simulink model "MHH_BUOI2_bai3"  (R2020b)
settings: Solver=VariableStepAuto  StartTime=0.0  StopTime=Sim_Time  RelTol=1e-3
values from neighbouring files (symbols this model uses):
  Cn = 8280    [Bai3_4.mat]
  I = 2.3    [Bai3_4.mat]
  OCV = [2.4 2.86404 3.33456 3.47124 3.5586 3.62364 3.6762 3.72036 3.7584 3.7902 3.81708 3.83568 ... (101 elements, 101x1)]    [Bai3_4.mat]    (also in bai4.mat)
  R_Discharge = [0.14 0.129 0.12383 0.09468 0.08038 0.07532 0.07257 0.07059 0.06894 0.06707 0.06498 0.06256 ... (101 elements, 101x1)]    [Bai3_4.mat]
  SOC = [0 0.01 0.02 0.03 0.04 0.05 0.06 0.07 0.08 0.09 0.1 0.11 ... (101 elements, 101x1)]    [Bai3_4.mat]    (also in bai4.mat)
settings Model: Creator=John Andrew  LastModifiedBy=John Andrew

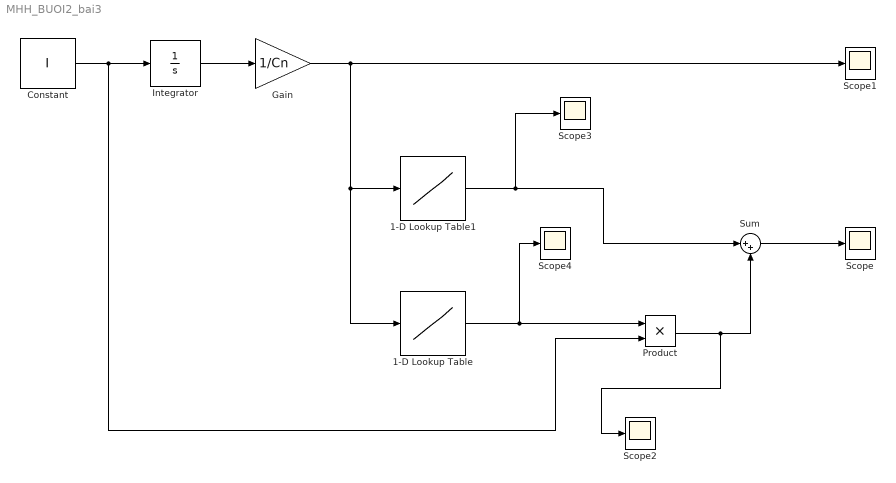
== system MHH_BUOI2_bai3 ==
  1-D Lookup Table : Lookup_n-D  NumberOfTableDimensions=1  BreakpointsForDimension1=SOC  Table=R_Discharge  InternalRulePriority=Speed  RndMeth=Simplest  InputSameDT=on
  1-D Lookup Table1 : Lookup_n-D  NumberOfTableDimensions=1  BreakpointsForDimension1=SOC  Table=OCV  InternalRulePriority=Speed  RndMeth=Simplest  InputSameDT=on
  Constant : Constant  Value=I
  Gain : Gain  Gain=1/Cn
  Integrator : Integrator
  Product : Product
  Scope{,1..4} (5 alike) : Scope
  Sum : Sum  Inputs=|++
  wires:
  Integrator/1 -> Gain/1
  Gain/1 -> 1-D Lookup Table/1, 1-D Lookup Table1/1, Scope1/1
  Constant/1 -> Product/2, Integrator/1
  1-D Lookup Table1/1 -> Scope3/1, Sum/1
  1-D Lookup Table/1 -> Scope4/1, Product/1
  Product/1 -> Scope2/1, Sum/2
  Sum/1 -> Scope/1
